simulink model "lseg"  (Simulink 6.6)
settings: Solver=ode45  StartTime=0.0  StopTime=Te  RelTol=1e-3
values from neighbouring files (symbols this model uses):
  C = [1 0 0 0;0 1 0 0;0 0 0 0;0 0 0 0]    [hseg.m]    (also in seg.m = [1 0 0 0])
  D = [0 0;0 0;eye(2)]    [hseg.m]
  F = Fl    [seg.m]
  ue = [0;0]    [seg.m]
undefined symbols (not defined in the file or in its folder): A, B, ye
libraries: cstblocks x1
settings Model: Creator=cscherer  LastModifiedBy=carsten
settings DebuggingCC: SignalResolutionControl=TryResolveAllWithWarning  MultiTaskDSMMsg=warning  MultiTaskCondExecSysMsg=none  StrictBusMsg=None
settings RTWCC: IncludeERTFirstTime=on

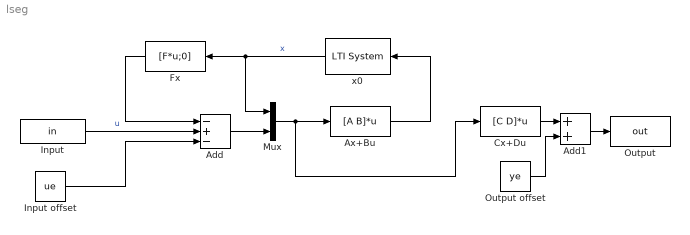
== system lseg ==
  Add : Sum  Inputs=-+-  OutScaling=2^-10
  Add1 : Sum  OutScaling=2^-10
  Ax+Bu : MATLABFcn  MATLABFcn=[A B]*u
  Cx+Du : MATLABFcn  MATLABFcn=[C D]*u
  Fx : MATLABFcn  Orientation=left  MATLABFcn=[F*u;0]
  Input : FromWorkspace  VariableName=in  SampleTime=0  OutputAfterFinalValue=Setting to zero
  Input offset : Constant  Value=ue
  Mux : Mux  Inputs=2
  Output : ToWorkspace  VariableName=out  SampleTime=-1  SaveFormat=Structure With Time
  Output offset : Constant  Value=ye
  x0 : cstblocks/LTI System  Orientation=left  SystemSampleTime=-1  sys=integrator  IC=x0
  wires:
  Mux/1 -> Ax+Bu/1, Cx+Du/1
  Ax+Bu/1 -> x0/1
  x0/1 -> Mux/1, Fx/1  "x"
  Add/1 -> Mux/2
  Add1/1 -> Output/1
  Cx+Du/1 -> Add1/1
  Output offset/1 -> Add1/2
  Input offset/1 -> Add/3
  Input/1 -> Add/2  "u"
  Fx/1 -> Add/1
